simulink model "Non_Linear_model"  (R2025b)
settings: Solver=VariableStepAuto  StartTime=0.0  StopTime=20  RelTol=1e-3
InitFcn:
  | load('drone_model_parameters.mat');
values from neighbouring files (symbols this model uses):
  g = 9.81    [drone_model_parameters.mat]
  J11 = 5.8286e-05    [drone_model_parameters.mat]
  J22 = 7.1691e-05    [drone_model_parameters.mat]
  J33 = 3e-05    [drone_model_parameters.mat]
  K2 = K2_sat    [untitled.m]
  K3 = K3_sat    [untitled.m]
  K4 = K4_sat    [untitled.m]
  K_T = 4.72e-08    [drone_model_parameters.mat]
  K_tau = 1.1393e-10    [drone_model_parameters.mat]
  K_u = 13840.4    [drone_model_parameters.mat]
  ki1 = ki1_sat    [untitled.m]
  ki2 = ki2_sat    [untitled.m]
  ki3 = ki3_sat    [untitled.m]
  ki4 = ki4_sat    [untitled.m]
  L = 0.0624    [drone_model_parameters.mat]
  m = 0.063    [drone_model_parameters.mat]
  omega0 = zeros(3,1)    [untitled.m]
  phi_ref = 0.5    [untitled.m]
  r_n0 = zeros(3,1)    [untitled.m]
  theta0 = zeros(3,1)    [untitled.m]
  u_imax = 500    [Q20_saturation_data.mat]    (also in drone_model_parameters.mat; untitled.m)
  v0 = zeros(3,1)    [untitled.m]
  x_ref = 2    [untitled.m]
  y_ref = 1    [untitled.m]
  z_ref = 0.5    [untitled.m]
undefined symbols (not defined in the file or in its folder): K1
libraries: matrix_library x1
settings Model: Creator=Lenovo  LastModifiedBy=joaom

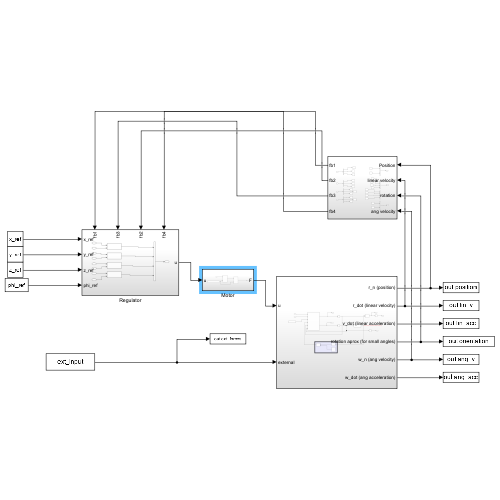
[thumbnail: Simulink's stored preview of the top-level diagram]
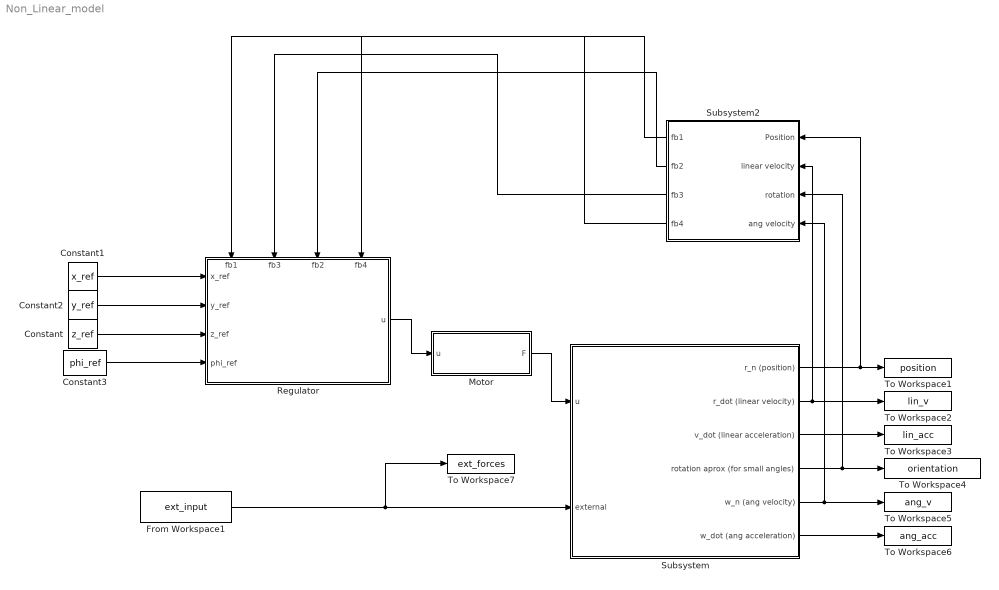
== system Non_Linear_model ==
  Constant : Constant  Value=z_ref
  Constant1 : Constant  Value=x_ref
  Constant2 : Constant  Value=y_ref
  Constant3 : Constant  Value=phi_ref
  From Workspace1 : FromWorkspace  VariableName=ext_input  SampleTime=0.01
  Motor : Subsystem
  Regulator : Subsystem
      settings: PortSchema="{\"entries\":[{\"content\":{\"sides\":[{\"content\":{\"connectorIds\":[\"In1\",\"In2\",\"In3\",\"In4\"]},\"type\":\"ConnectorPlacement.EquallySpacedRectSide\",\"uuid\":\"b017568b-8a8c-41ec-878a-07ad52499eb1\"},{\"content\":{\"connectorIds\":[\"Out1\"],\"side\":\"RIGHT\"},\"type\":\"ConnectorPlacement.EquallySpacedRectSide\",\"uuid\":\"018e7ed3-6d8e-4146-8286-a6e4e64e27eb\"},{\"content\":{\"connectorIds\":[\"In5\",\"In6\",\"In7\",\"In8\"],\"side\":\"TOP\"},\"type\":\"ConnectorPlacement.EquallySpacedRectSide\",\"uuid\":\"74bee916-3a13-46de-9b7b-1c6e20b8f68c\"}]},\"type\":\"ConnectorPlacement.EquallySpacedConnector\",\"uuid\":\"c4290e45-5abb-401a-ab88-e47e173bbe8b\"}],\"packageUris\":[\"http://schema.mathworks.com/mf0/Connector/R2020b\"],\"version\":\"1.0\"}"
  Subsystem : Subsystem
  Subsystem2 : Subsystem
  To Workspace1 : ToWorkspace  VariableName=position  SaveFormat=Timeseries  SampleTime=-1
  To Workspace2 : ToWorkspace  VariableName=lin_v  SaveFormat=Timeseries  SampleTime=-1
  To Workspace3 : ToWorkspace  VariableName=lin_acc  SaveFormat=Timeseries  SampleTime=-1
  To Workspace4 : ToWorkspace  VariableName=orientation  SaveFormat=Timeseries  SampleTime=-1
  To Workspace5 : ToWorkspace  VariableName=ang_v  SaveFormat=Timeseries  SampleTime=-1
  To Workspace6 : ToWorkspace  VariableName=ang_acc  SaveFormat=Timeseries  SampleTime=-1
  To Workspace7 : ToWorkspace  VariableName=ext_forces  SaveFormat=Timeseries  SampleTime=-1
  wires:
  Subsystem/1(r_n (position)) -> Subsystem2/1(Position), To Workspace1/1
  From Workspace1/1 -> To Workspace7/1, Subsystem/2(external)
  Subsystem/2(r_dot (linear velocity)) -> Subsystem2/2(linear velocity), To Workspace2/1
  Subsystem/4(rotation aprox (for small angles)) -> Subsystem2/3(rotation), To Workspace4/1
  Subsystem/5(w_n (ang velocity)) -> Subsystem2/4(ang velocity), To Workspace5/1
  Subsystem/6(w_dot (ang acceleration)) -> To Workspace6/1
  Subsystem/3(v_dot (linear acceleration)) -> To Workspace3/1
  Subsystem2/1(fb1) -> Regulator/5(fb1)
  Subsystem2/4(fb4) -> Regulator/8(fb4)
  Constant3/1 -> Regulator/4(phi_ref)
  Constant/1 -> Regulator/3(z_ref)
  Constant2/1 -> Regulator/2(y_ref)
  Constant1/1 -> Regulator/1(x_ref)
  Subsystem2/2(fb2) -> Regulator/7(fb2)
  Subsystem2/3(fb3) -> Regulator/6(fb3)
  Regulator/1(u) -> Motor/1(u)
  Motor/1(F) -> Subsystem/1(u)

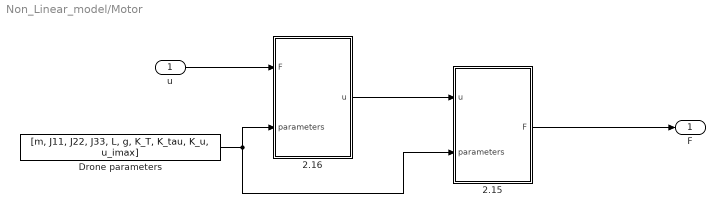
== system Non_Linear_model/Motor ==
  u : Inport
  2.15 : MATLAB Function  TreatAsAtomicUnit=on
  2.16 : MATLAB Function  TreatAsAtomicUnit=on
  Drone parameters : Constant  Value=[m, J11, J22, J33, L, g, K_T, K_tau, K_u, u_imax]
  F : Outport
  wires:
  2.15/1(F) -> F/1
  2.16/1(u) -> 2.15/1(u)
  Drone parameters/1 -> 2.16/2(parameters), 2.15/2(parameters)
  u/1 -> 2.16/1(F)

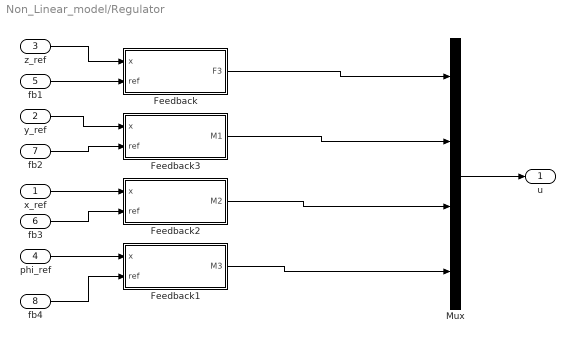
== system Non_Linear_model/Regulator ==
  x_ref : Inport
  y_ref : Inport  Port=2
  z_ref : Inport  Port=3
  phi_ref : Inport  Port=4
  fb1 : Inport  Port=5
  fb3 : Inport  Port=6
  fb2 : Inport  Port=7
  fb4 : Inport  Port=8
  Feedback : Subsystem
  Feedback1 : Subsystem
  Feedback2 : Subsystem
  Feedback3 : Subsystem
  Mux : Mux
  u : Outport
  wires:
  Feedback2/1(M2) -> Mux/3
  Feedback3/1(M1) -> Mux/2
  Feedback/1(F3) -> Mux/1
  Feedback1/1(M3) -> Mux/4
  Mux/1 -> u/1
  x_ref/1 -> Feedback2/1(x)
  y_ref/1 -> Feedback3/1(x)
  z_ref/1 -> Feedback/1(x)
  phi_ref/1 -> Feedback1/1(x)
  fb1/1 -> Feedback/2(ref)
  fb2/1 -> Feedback3/2(ref)
  fb3/1 -> Feedback2/2(ref)
  fb4/1 -> Feedback1/2(ref)

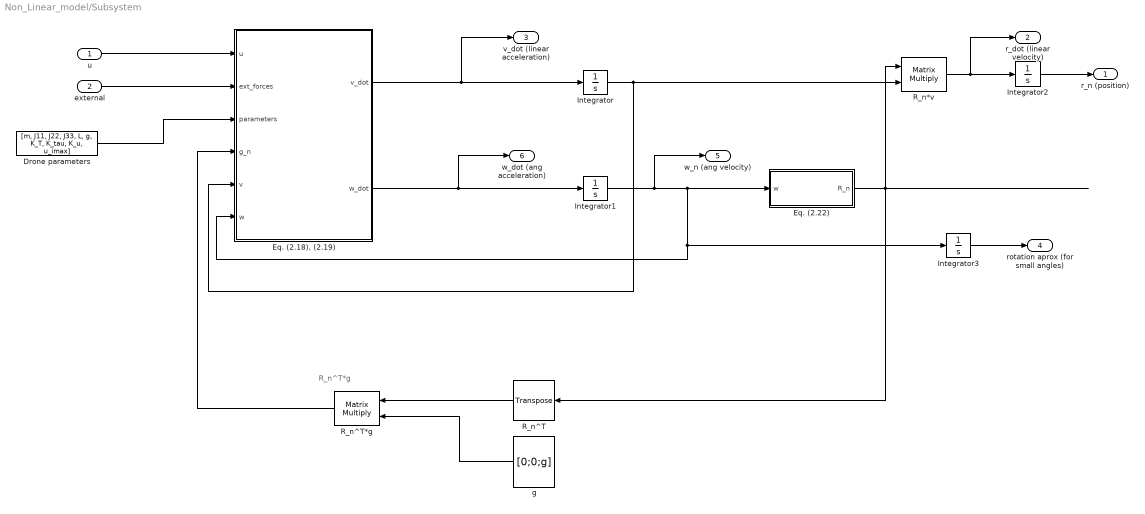
== system Non_Linear_model/Subsystem ==
  note: R_n^T*g
  u : Inport
  external : Inport  Port=2
  Drone parameters : Constant  Value=[m, J11, J22, J33, L, g, K_T, K_tau, K_u, u_imax]
  "Eq. (2.18), (2.19) " : MATLAB Function  TreatAsAtomicUnit=on
  Eq. (2.22) : Subsystem
  Integrator : Integrator  InitialCondition=v0
  Integrator1 : Integrator  InitialCondition=omega0
  Integrator2 : Integrator  InitialCondition=r_n0
  Integrator3 : Integrator  InitialCondition=theta0
  R_n*v : Product  Multiplication=Matrix(*)
  R_n^T : matrix_library/Transpose
  R_n^T*g : Product  Multiplication=Matrix(*)
  g : Constant  Value=[0;0;g]  VectorParams1D=off
  r_n (position) : Outport
  r_dot (linear velocity) : Outport  Port=2
  v_dot (linear acceleration) : Outport  Port=3
  rotation aprox (for small angles) : Outport  Port=4
  w_n (ang velocity) : Outport  Port=5
  w_dot (ang acceleration) : Outport  Port=6
  wires:
  u/1 -> "Eq. (2.18), (2.19) "/1(u)
  external/1 -> "Eq. (2.18), (2.19) "/2(ext_forces)
  Drone parameters/1 -> "Eq. (2.18), (2.19) "/3(parameters)
  Eq. (2.22)/1(R_n) -> R_n*v/1, R_n^T/1
  R_n*v/1 -> r_dot (linear velocity)/1, Integrator2/1
  Integrator2/1 -> r_n (position)/1
  "Eq. (2.18), (2.19) "/1(v_dot) -> v_dot (linear acceleration)/1, Integrator/1
  "Eq. (2.18), (2.19) "/2(w_dot) -> w_dot (ang acceleration)/1, Integrator1/1
  Integrator/1 -> "Eq. (2.18), (2.19) "/5(v), R_n*v/2
  Integrator1/1 -> w_n (ang velocity)/1, Eq. (2.22)/1(w), "Eq. (2.18), (2.19) "/6(w), Integrator3/1
  Integrator3/1 -> rotation aprox (for small angles)/1
  R_n^T/1 -> R_n^T*g/1
  g/1 -> R_n^T*g/2
  R_n^T*g/1 -> "Eq. (2.18), (2.19) "/4(g_n)

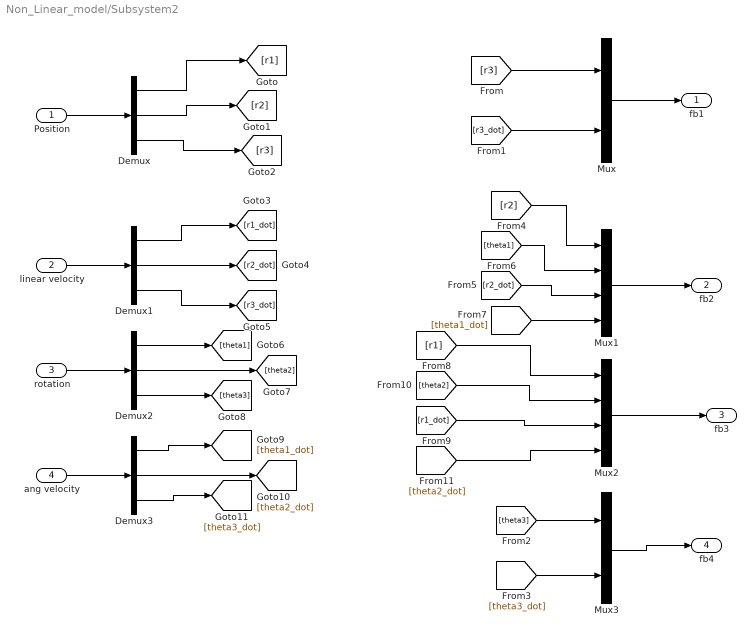
== system Non_Linear_model/Subsystem2 ==
  Position : Inport
  linear velocity : Inport  Port=2
  rotation : Inport  Port=3
  ang velocity : Inport  Port=4
  Demux{,1..3} (4 alike) : Demux  Outputs=3
  Mux : Mux  Inputs=2
  Mux1 : Mux
  Mux2 : Mux
  Mux3 : Mux  Inputs=2
  fb1 : Outport
  fb2 : Outport  Port=2
  fb3 : Outport  Port=3
  fb4 : Outport  Port=4
  wires:
  linear velocity/1 -> Demux1/1
  Position/1 -> Demux/1
  rotation/1 -> Demux2/1
  ang velocity/1 -> Demux3/1
  Demux/1 -> [r1]
  Demux/2 -> [r2]
  Demux/3 -> [r3]
  Demux1/3 -> [r3_dot]
  Demux1/1 -> [r1_dot]
  Demux1/2 -> [r2_dot]
  Demux2/3 -> [theta3]
  Demux2/2 -> [theta2]
  Demux2/1 -> [theta1]
  [r3_dot] -> Mux/2
  [r3] -> Mux/1
  Mux3/1 -> fb4/1
  Mux2/1 -> fb3/1
  Mux1/1 -> fb2/1
  Mux/1 -> fb1/1
  Demux3/3 -> [theta3_dot]
  Demux3/2 -> [theta2_dot]
  Demux3/1 -> [theta1_dot]
  [theta3_dot] -> Mux3/2
  [theta3] -> Mux3/1
  [r2] -> Mux1/1
  [r2_dot] -> Mux1/3
  [theta1] -> Mux1/2
  [theta1_dot] -> Mux1/4
  [theta2_dot] -> Mux2/4
  [r1] -> Mux2/1
  [r1_dot] -> Mux2/3
  [theta2] -> Mux2/2

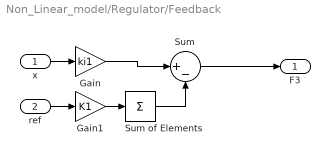
== system Non_Linear_model/Regulator/Feedback ==
  x : Inport
  ref : Inport  Port=2
  Gain : Gain  Gain=ki1
  Gain1 : Gain  Gain=K1
  Sum : Sum  Inputs=|+-
  Sum of Elements : Sum  Inputs=+
  F3 : Outport
  wires:
  x/1 -> Gain/1
  ref/1 -> Gain1/1
  Gain1/1 -> Sum of Elements/1
  Sum/1 -> F3/1
  Gain/1 -> Sum/1
  Sum of Elements/1 -> Sum/2

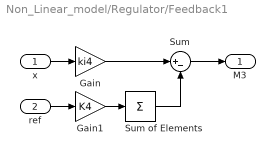
== system Non_Linear_model/Regulator/Feedback1 ==
  x : Inport
  ref : Inport  Port=2
  Gain : Gain  Gain=ki4
  Gain1 : Gain  Gain=K4
  Sum : Sum  Inputs=|+-
  Sum of Elements : Sum  Inputs=+
  M3 : Outport
  wires:
  x/1 -> Gain/1
  ref/1 -> Gain1/1
  Gain1/1 -> Sum of Elements/1
  Gain/1 -> Sum/1
  Sum of Elements/1 -> Sum/2
  Sum/1 -> M3/1

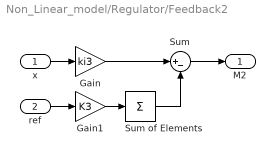
== system Non_Linear_model/Regulator/Feedback2 ==
  x : Inport
  ref : Inport  Port=2
  Gain : Gain  Gain=ki3
  Gain1 : Gain  Gain=K3
  Sum : Sum  Inputs=|+-
  Sum of Elements : Sum  Inputs=+
  M2 : Outport
  wires:
  x/1 -> Gain/1
  ref/1 -> Gain1/1
  Gain1/1 -> Sum of Elements/1
  Gain/1 -> Sum/1
  Sum of Elements/1 -> Sum/2
  Sum/1 -> M2/1

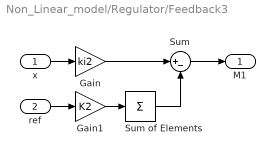
== system Non_Linear_model/Regulator/Feedback3 ==
  x : Inport
  ref : Inport  Port=2
  Gain : Gain  Gain=ki2
  Gain1 : Gain  Gain=K2
  Sum : Sum  Inputs=|+-
  Sum of Elements : Sum  Inputs=+
  M1 : Outport
  wires:
  x/1 -> Gain/1
  ref/1 -> Gain1/1
  Gain1/1 -> Sum of Elements/1
  Gain/1 -> Sum/1
  Sum of Elements/1 -> Sum/2
  Sum/1 -> M1/1

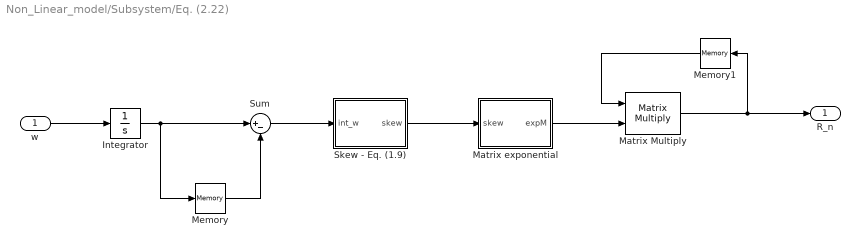
== system Non_Linear_model/Subsystem/Eq. (2.22) ==
  w : Inport
  Integrator : Integrator  InitialCondition=[0;0;0]
  Matrix Multiply : Product  Multiplication=Matrix(*)
  Matrix exponential : MATLAB Function  TreatAsAtomicUnit=on
  Memory : Memory  InitialCondition=[0 0 0]
  Memory1 : Memory  InitialCondition=eye(3)
  Skew - Eq. (1.9) : MATLAB Function  TreatAsAtomicUnit=on
  Sum : Sum  Inputs=|+-
  R_n : Outport
  wires:
  w/1 -> Integrator/1
  Integrator/1 -> Memory/1, Sum/1
  Memory/1 -> Sum/2
  Sum/1 -> Skew - Eq. (1.9)/1(int_w)
  Skew - Eq. (1.9)/1(skew) -> Matrix exponential/1(skew)
  Matrix exponential/1(expM) -> Matrix Multiply/2
  Matrix Multiply/1 -> Memory1/1, R_n/1
  Memory1/1 -> Matrix Multiply/1

== matlab function Non_Linear_model/Subsystem/Eq. (2.22)/Skew - Eq. (1.9) ==
  data: int_w input; skew output
function skew = fcn(int_w)

skew = [0 -int_w(3) int_w(2); int_w(3) 0 -int_w(1); -int_w(2) int_w(1) 0];

end

== matlab function Non_Linear_model/Subsystem/Eq. (2.18), (2.19)  ==
  data: u input; ext_forces input; parameters input; g_n input; v input size=3; w input size=3; v_dot output size=3; w_dot output size=3
function [v_dot, w_dot] = fcn(u, ext_forces, parameters, g_n, v, w)
% Implements Equations 2.18 and 2.19 from the quadcopter dynamics notes
%
% Inputs:
%   u           - control inputs [F3; M1; M2; M3]
%   ext_forces  - external force perturbations [F1ext; F2ext; F3ext] in body frame
%   parameters  - drone parameters [m; J11; J22; J33]
%   g_n         - gravity vector projected in body frame [g1; g2; g3]
%   v           - linear velocity in body frame [v1; v2; v3]
%   w           - angular velocity in body frame [w1; w2; w3]
%
% Outputs:
%   v_dot       - linear acceleration in body frame [v1_dot; v2_dot; v3_dot]
%   w_dot       - angular acceleration in body frame [w1_dot; w2_dot; w3_dot]

% ── Unpack parameters ─────────────────────────────────────────────────────
m   = parameters(1);
J11 = parameters(2);
J22 = parameters(3);
J33 = parameters(4);

% ── Unpack control inputs ─────────────────────────────────────────────────
F3 = u(1) - m * g_n(3);
M1 = u(2);
M2 = u(3);
M3 = u(4);

% ── Unpack external forces ────────────────────────────────────────────────
F1_ext = ext_forces(1);
F2_ext = ext_forces(2);
F3_ext = ext_forces(3);


% ── Linear acceleration - Eq. 2.18 ───────────────────────────────────────
% v_dot = Coriolis + thrust/ext forces + gravity projection
v_dot_1 = (v(2)*w(3) - v(3)*w(2)) + (F1_ext/m) + g_n(1);
v_dot_2 = (v(3)*w(1) - v(1)*w(3)) + (F2_ext/m) + g_n(2);
v_dot_3 = (v(1)*w(2) - v(2)*w(1)) + (F3/m) + (F3_ext/m) + g_n(3);

% ── Angular acceleration - Eq. 2.19 ──────────────────────────────────────
% w_dot = gyroscopic terms + applied moments
w_dot_1 = ((J22-J33)/J11) * w(2)*w(3) + M1/J11;
w_dot_2 = ((J33-J11)/J22) * w(1)*w(3) + M2/J22;
w_dot_3 = ((J11-J22)/J33) * w(1)*w(2) + M3/J33;

% ── Pack outputs ──────────────────────────────────────────────────────────
v_dot = [v_dot_1; v_dot_2; v_dot_3];
w_dot = [w_dot_1; w_dot_2; w_dot_3];

== matlab function Non_Linear_model/Subsystem/Eq. (2.22)/Matrix exponential ==
  data: skew input; expM output
function expM = fcn(skew)

expM = expm(skew);

== matlab function Non_Linear_model/Motor/2.16 ==
  data: F input; u output; parameters input
function u = fcn(F, parameters)

L=parameters(5);
K_T=parameters(7);
K_tau=parameters(8);
K_u=parameters(9);
u_imax=parameters(10);

C_pi_4 = cos(pi/4);

T_matrix = [
    -1/K_T,   (1/(K_T * L * C_pi_4)),  (1/(K_T * L * C_pi_4)),  -1/K_tau;
    -1/K_T,  -1/(K_T * L * C_pi_4),   (1/(K_T * L * C_pi_4)),  1/K_tau;
    -1/K_T,   (-1/(K_T * L * C_pi_4)),  -1/(K_T * L * C_pi_4),  -1/K_tau;
    -1/K_T,  1/(K_T * L * C_pi_4),   -1/(K_T * L * C_pi_4),   1/K_tau
];

u = (1 / (4 * K_u)) * T_matrix * F;
u(u > u_imax) = u_imax;

== matlab function Non_Linear_model/Motor/2.15 ==
  data: u input; parameters input; F output
function F = fcn(u, parameters)

L=parameters(5);
K_T=parameters(7);
K_tau=parameters(8);
K_u=parameters(9);

C_pi_4 = cos(pi/4);

K_matrix = [
    -K_T,  -K_T,  -K_T,  -K_T;
     L*C_pi_4*K_T, -L*C_pi_4*K_T, -L*C_pi_4*K_T,  L*C_pi_4*K_T;
     L*C_pi_4*K_T,  L*C_pi_4*K_T, -L*C_pi_4*K_T, -L*C_pi_4*K_T;
    -K_tau,  K_tau, -K_tau,  K_tau
];


% Compute the force-moment vector
F = K_u * K_matrix * u;
